simulink model "Pokus05_Instruction_Decoder"  (Simulink 8.1)
settings: Solver=ode45  StartTime=0.0  StopTime=10.0  RelTol=1e-3
undefined symbols (not defined in the file): sigbuilder_block
libraries: Common_Library x4, simulink_extras x3, commutil2 x1
settings Model: Creator=uzivatel  LastModifiedBy=uzivatel
settings DataIOCC: SignalLoggingSaveFormat=Dataset
settings OptimizationCC: ExpressionDepthLimit=128
settings DebuggingCC: FcnCallInpInsideContextMsg=EnableAllAsError
settings GRTTargetCC: CombineOutputUpdateFcns=on  GRTInterface=off

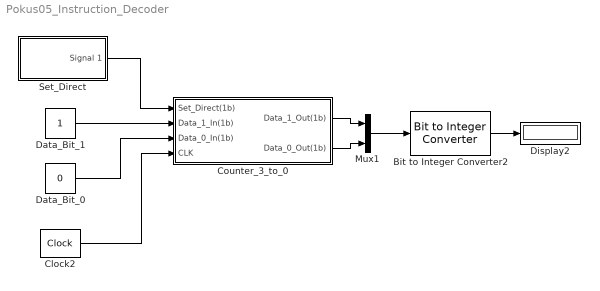
== system Pokus05_Instruction_Decoder ==
  Bit to Integer Converter2 : commutil2/Bit to Integer Converter  nbits=2  bitOrder=MSB first  signedOutputValues=Unsigned  outDtype=uint8  outDtypeSigned=Inherit via internal rule
  Clock2 : simulink_extras/Flip Flops/Clock  period=1
  Counter_3_to_0 : Subsystem
  Data_Bit_0 : Constant  Value=0
  Data_Bit_1 : Constant
  Display2 : Display
  Mux1 : Mux  Inputs=2
  Set_Direct : Subsystem  Tag=STV Subsys  LoadFcn=sigbuilder_block('load');  StartFcn=sigbuilder_block('start');  StopFcn=sigbuilder_block('stop');  ClipboardFcn=sigbuilder_block('clipboard');  mask(Sigbuilder block){}
      mask help: Simulink:masks:SigbuilderBlock_MD
      mask init:
      | if ~strcmp(get_param(bdroot(gcbh),'SimulationStatus'),'stopped') tuvar = sigbuilder_block('maskInit'); end
      settings: CopyFcn=sigbuilder_block('copy');  DeleteFcn=sigbuilder_block('delete');  ModelCloseFcn=sigbuilder_block('modelClose');  PreSaveFcn=sigbuilder_block('preSave');  PauseFcn=sigbuilder_block('pause');  ContinueFcn=sigbuilder_block('continue');  NameChangeFcn=sigbuilder_block('namechange');  OpenFcn=sigbuilder_block('open',[437.6 199.2 550.4 400 ]);  CloseFcn=sigbuilder_block('close');
      mask Display: plot(0, 0, 100, 100,[2, 2, 32, 32, 2], [68, 8, 8, 68, 68],[32, 2], [38, 38], [32, 19, 2],[53, 60, 44], [32, 17, 17, 2],[16, 16, 31, 31]);txt = getActiveGroup(gcbh);text(2, 100, txt,'verticalAlignment', 'top');
  wires:
  Mux1/1 -> Bit to Integer Converter2/1
  Bit to Integer Converter2/1 -> Display2/1
  Counter_3_to_0/1(Data_1_Out(1b)) -> Mux1/1
  Counter_3_to_0/2(Data_0_Out(1b)) -> Mux1/2
  Set_Direct/1(Signal 1) -> Counter_3_to_0/1(Set_Direct(1b))
  Data_Bit_0/1 -> Counter_3_to_0/3(Data_0_In(1b))
  Data_Bit_1/1 -> Counter_3_to_0/2(Data_1_In(1b))
  Clock2/1 -> Counter_3_to_0/4(CLK)

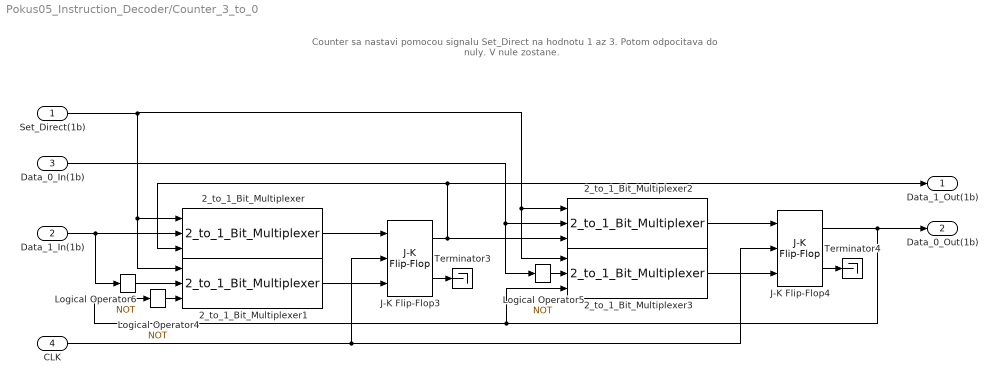
== system Pokus05_Instruction_Decoder/Counter_3_to_0 ==
  note: Counter sa nastavi pomocou signalu Set_Direct na hodnotu 1 az 3.
      | Potom odpocitava do nuly. V nule zostane.
  Set_Direct(1b) : Inport
  Data_1_In(1b) : Inport  Port=2
  Data_0_In(1b) : Inport  Port=3
  CLK : Inport  Port=4
  2_to_1_Bit_Multiplexer{,1..3} (4 alike) : Common_Library/Multiplexers/2_to_1_Bit_Multiplexer
  J-K Flip-Flop3 : simulink_extras/Flip Flops/J-K Flip-Flop  initial_condition=0
  J-K Flip-Flop4 : simulink_extras/Flip Flops/J-K Flip-Flop  initial_condition=0
  Logical Operator4 : Logic  Operator=NOT  IconShape=distinctive  AllPortsSameDT=off  OutDataTypeStr=boolean
  Logical Operator5 : Logic  Operator=NOT  IconShape=distinctive  AllPortsSameDT=off  OutDataTypeStr=boolean
  Logical Operator6 : Logic  Operator=NOT  IconShape=distinctive  AllPortsSameDT=off  OutDataTypeStr=boolean
  Terminator3 : Terminator
  Terminator4 : Terminator
  Data_1_Out(1b) : Outport
  Data_0_Out(1b) : Outport  Port=2
  wires:
  J-K Flip-Flop4/2 -> Terminator4/1
  J-K Flip-Flop3/1 -> Data_1_Out(1b)/1, 2_to_1_Bit_Multiplexer/3, 2_to_1_Bit_Multiplexer2/3
  Logical Operator4/1 -> 2_to_1_Bit_Multiplexer1/3
  J-K Flip-Flop4/1 -> Data_0_Out(1b)/1, 2_to_1_Bit_Multiplexer3/3, Logical Operator4/1
  CLK/1 -> J-K Flip-Flop4/2, J-K Flip-Flop3/2
  J-K Flip-Flop3/2 -> Terminator3/1
  Logical Operator6/1 -> 2_to_1_Bit_Multiplexer1/2
  2_to_1_Bit_Multiplexer/1 -> J-K Flip-Flop3/1
  2_to_1_Bit_Multiplexer1/1 -> J-K Flip-Flop3/3
  Data_1_In(1b)/1 -> Logical Operator6/1, 2_to_1_Bit_Multiplexer/2
  Set_Direct(1b)/1 -> 2_to_1_Bit_Multiplexer1/1, 2_to_1_Bit_Multiplexer/1, 2_to_1_Bit_Multiplexer3/1, 2_to_1_Bit_Multiplexer2/1
  Data_0_In(1b)/1 -> 2_to_1_Bit_Multiplexer2/2, Logical Operator5/1
  Logical Operator5/1 -> 2_to_1_Bit_Multiplexer3/2
  2_to_1_Bit_Multiplexer2/1 -> J-K Flip-Flop4/1
  2_to_1_Bit_Multiplexer3/1 -> J-K Flip-Flop4/3

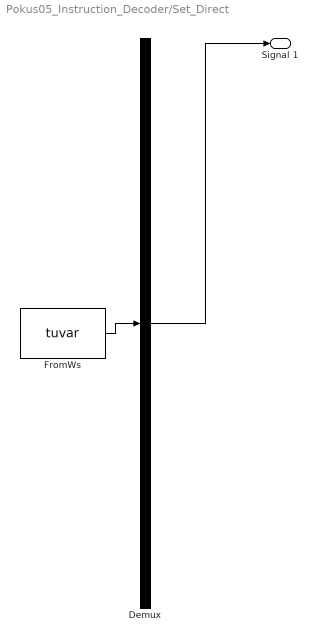
== system Pokus05_Instruction_Decoder/Set_Direct ==
  Demux : Demux  Tag=STV Demux  Outputs=1
  FromWs : FromWorkspace  Tag=STV FromWs  VariableName=tuvar  SampleTime=0  SigBuilderData=DataTag0  VnvData=DataTag1
      SigBuilderData=|
      | common.afterFinalStr = 'Extrapolate'
      | common.sampleTime = 0
      | dataSet.timeRange = [0 10]
      | dataSet.name = 'Group 1'
      | sbobj.Groups.Name = 'Group 1'
      | sbobj.Groups.Signals.Name = 'Signal 1'
      | sbobj.Groups.Signals.XData = [0 2 2 3 3 10]
      | sbobj.Groups.Signals.YData = [0 0 1 1 0 0]
  Signal 1 : Outport  Tag=STV Outport
  wires:
  Demux/1 -> Signal 1/1
  FromWs/1 -> Demux/1
